simulink model "amortiguador"  (R2023a)
settings: Solver=VariableStepAuto  StartTime=0.0  StopTime=10  MaxStep=0.01  RelTol=1e-3
model workspace (MAT data in the model file):
  Amp1 = 1
  Amp2 = 0.5
  Amp3 = 0.75
  Amp4 = 0.3
  Bias1 = 0.1
  Bias2 = 0.1
  Bias3 = 0.6
  Cc = 30
  Freq1 = 2
  Freq2 = 3
  Freq3 = 2
  Kc = 20
  Kr = 700
  Mc = 60
  Mr = 12
  Phase1 = 0.5
  Phase2 = 3
  Phase3 = 6
libraries: SignalEditorBlockLib x1
settings Model: Creator=santi  LastModifiedBy=santi

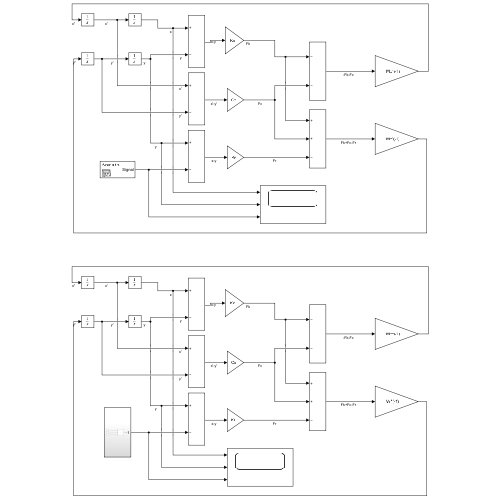
[thumbnail: Simulink's stored preview of the top-level diagram]
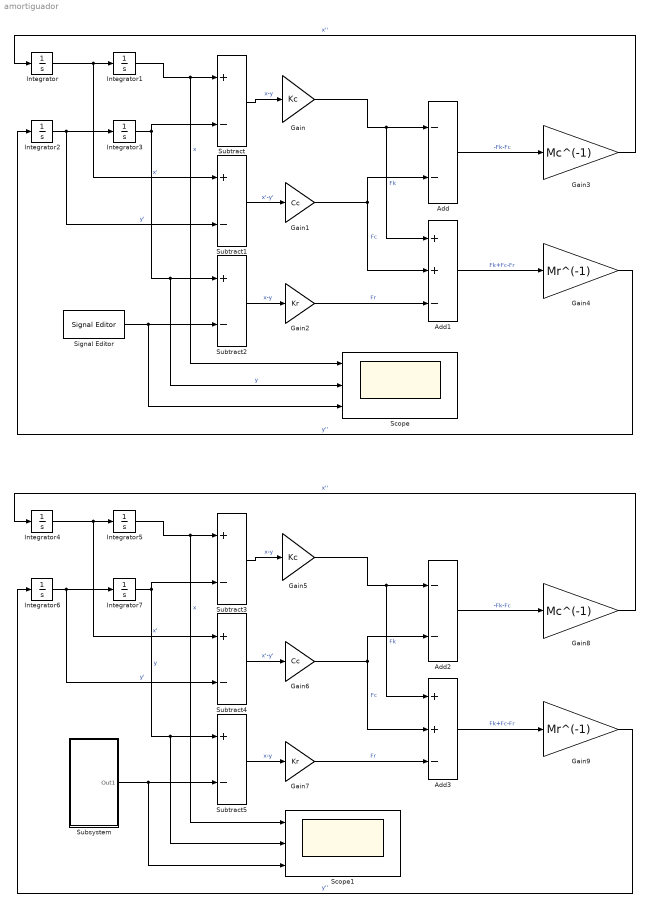
== system amortiguador ==
  Add : Sum  Inputs=--
  Add1 : Sum  Inputs=++-
  Add2 : Sum  Inputs=--
  Add3 : Sum  Inputs=++-
  Gain : Gain  Gain=Kc
  Gain1 : Gain  Gain=Cc
  Gain2 : Gain  Gain=Kr
  Gain3 : Gain  Gain=Mc^(-1)
  Gain4 : Gain  Gain=Mr^(-1)
  Gain5 : Gain  Gain=Kc
  Gain6 : Gain  Gain=Cc
  Gain7 : Gain  Gain=Kr
  Gain8 : Gain  Gain=Mc^(-1)
  Gain9 : Gain  Gain=Mr^(-1)
  Integrator{,1..7} (8 alike) : Integrator
  Scope : Scope  NumInputPorts=3
  Scope1 : Scope  NumInputPorts=3
  Signal Editor : SignalEditorBlockLib/Signal Editor  FileName=Terreno.mat  ActiveScenario=Scenario  ActiveSignal=Signal  IsBus=off  OutputBusObjectStr=Bus: BusObject  SampleTime=0  Interpolate=off  ZeroCross=off  OutputAfterFinalValue=Setting to zero  Unit=inherit  PreserveSignalName=on  ApplySigPropsToAllScenarios=on
  Subsystem : Subsystem
  Subtract{,1..5} (6 alike) : Sum  Inputs=+-
  wires:
  Integrator/1 -> Subtract1/1, Integrator1/1  "x'"
  Gain3/1 -> Integrator/1  "x''"
  Integrator1/1 -> Scope/1, Subtract/1  "x"
  Integrator3/1 -> Scope/2, Subtract2/1, Subtract/2  "y"
  Gain4/1 -> Integrator2/1  "y''"
  Integrator2/1 -> Subtract1/2, Integrator3/1  "y'"
  Subtract/1 -> Gain/1  "x-y"
  Gain/1 -> Add1/1, Add/1  "Fk"
  Subtract1/1 -> Gain1/1  "x'-y'"
  Gain1/1 -> Add1/2, Add/2  "Fc"
  Subtract2/1 -> Gain2/1  "x-y"
  Gain2/1 -> Add1/3  "Fr"
  Add/1 -> Gain3/1  "-Fk-Fc"
  Add1/1 -> Gain4/1  "Fk+Fc-Fr"
  Signal Editor/1 -> Scope/3, Subtract2/2
  Subsystem/1(Out1) -> Subtract5/2, Scope1/3
  Add3/1 -> Gain9/1  "Fk+Fc-Fr"
  Add2/1 -> Gain8/1  "-Fk-Fc"
  Gain7/1 -> Add3/3  "Fr"
  Subtract5/1 -> Gain7/1  "x-y"
  Gain6/1 -> Add2/2, Add3/2  "Fc"
  Subtract4/1 -> Gain6/1  "x'-y'"
  Gain5/1 -> Add2/1, Add3/1  "Fk"
  Subtract3/1 -> Gain5/1  "x-y"
  Integrator6/1 -> Integrator7/1, Subtract4/2  "y'"
  Gain9/1 -> Integrator6/1  "y''"
  Integrator7/1 -> Subtract3/2, Subtract5/1, Scope1/2  "y"
  Integrator5/1 -> Subtract3/1, Scope1/1  "x"
  Gain8/1 -> Integrator4/1  "x''"
  Integrator4/1 -> Integrator5/1, Subtract4/1  "x'"

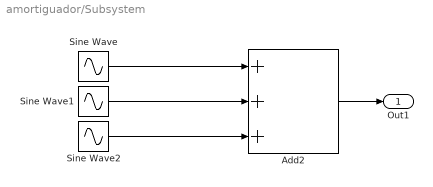
== system amortiguador/Subsystem ==
  Add2 : Sum  Inputs=+++
  Sine Wave : Sin  Amplitude=Amp1  Bias=Bias1  Frequency=Freq1  Phase=Phase1  SampleTime=0
  Sine Wave1 : Sin  Amplitude=Amp2  Bias=Bias2  Frequency=Freq2  Phase=Phase2  SampleTime=0
  Sine Wave2 : Sin  Amplitude=Amp3  Bias=Bias3  Frequency=Freq3  Phase=Phase3  SampleTime=0
  Out1 : Outport
  wires:
  Sine Wave1/1 -> Add2/2
  Sine Wave/1 -> Add2/1
  Sine Wave2/1 -> Add2/3
  Add2/1 -> Out1/1
